simulink model "lqr_linear"  (R2018a)
settings: Solver=FixedStepAuto  StartTime=0.0  StopTime=10  FixedStep=0.001  RelTol=1e-3
values from neighbouring files (symbols this model uses):
  A_dc = [(A_d-B_d*K_d)]    [Project_LQR.m]
  Ac = [(A-B*K)]    [Project_LQR.m]
  B_dc = [B_d]    [Project_LQR.m]
  Bc = [B]    [Project_LQR.m]
  C_dc = [C_d]    [Project_LQR.m]
  Cc = [C]    [Project_LQR.m]
  D_dc = [D_d]    [Project_LQR.m]
  Dc = [D]    [Project_LQR.m]
  Nbar = Nu + K*Nx    [Project_LQR.m]
  Nbar_d = K_d(3)    [Project_LQR.m]
  R_Wheel = 0.04    [Project_LQR.m]    (also in Project_PID.m)
libraries: simulink x5
settings Model: Creator=adios  LastModifiedBy=adios

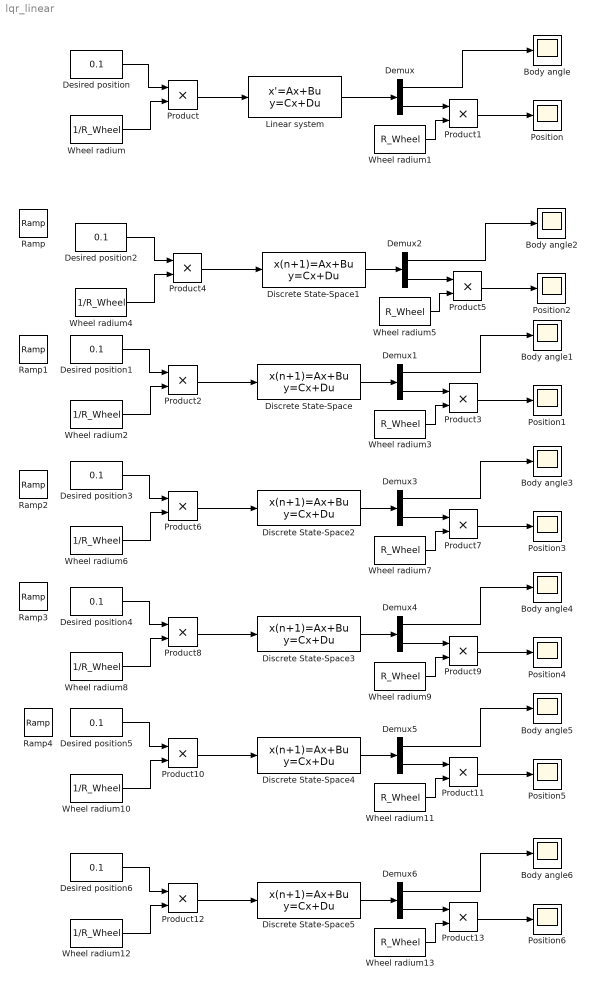
== system lqr_linear ==
  Body angle{,1..6} (7 alike) : Scope
  Demux{,1..6} (7 alike) : Demux  Outputs=2
  Desired position{,1..6} (7 alike) : Constant  Value=0.1
  Discrete State-Space : DiscreteStateSpace  A=A_dc  B=B_dc*Nbar_d  C=C_dc  D=D_dc  InitialCondition=[0 0 0 0]  SampleTime=0.02
  Discrete State-Space1 : DiscreteStateSpace  A=A_dc  B=B_dc*Nbar_d  C=C_dc  D=D_dc  InitialCondition=[0 0 0 0]  SampleTime=0.01
  Discrete State-Space2 : DiscreteStateSpace  A=A_dc  B=B_dc*Nbar_d  C=C_dc  D=D_dc  InitialCondition=[0 0 0 0]  SampleTime=0.04
  Discrete State-Space3 : DiscreteStateSpace  A=A_dc  B=B_dc*Nbar_d  C=C_dc  D=D_dc  InitialCondition=[0 0 0 0]  SampleTime=0.06
  Discrete State-Space4 : DiscreteStateSpace  A=A_dc  B=B_dc*Nbar_d  C=C_dc  D=D_dc  InitialCondition=[0 0 0 0]  SampleTime=0.08
  Discrete State-Space5 : DiscreteStateSpace  A=A_dc  B=B_dc*Nbar_d  C=C_dc  D=D_dc  InitialCondition=[0 0 0 0]  SampleTime=0.1
  Linear system : StateSpace  A=Ac  B=Bc*Nbar  C=Cc  D=Dc  InitialCondition=[0 0 0 0]  ContinuousStateAttributes=['theta' 'theta_dot' 'phi' 'phi_dot']
  Position{,1..6} (7 alike) : Scope
  Product{,1..13} (14 alike) : Product
  Ramp : simulink/Sources/Ramp  slope=0.1  start=0  InitialOutput=0
  Ramp1 : simulink/Sources/Ramp  slope=0.3  start=0  InitialOutput=0
  Ramp2 : simulink/Sources/Ramp  slope=0.5  start=0  InitialOutput=0
  Ramp3 : simulink/Sources/Ramp  slope=0.75  start=0  InitialOutput=0
  Ramp4 : simulink/Sources/Ramp  slope=1  start=0  InitialOutput=0
  Wheel radium{,2,4,6,8,10,12} (7 alike) : Constant  Value=1/R_Wheel
  Wheel radium{1,3,5,7,9,11,13} (7 alike) : Constant  Value=R_Wheel
  wires:
  Linear system/1 -> Demux/1
  Desired position/1 -> Product/1
  Wheel radium/1 -> Product/2
  Product/1 -> Linear system/1
  Demux/1 -> Body angle/1
  Demux/2 -> Product1/1
  Wheel radium1/1 -> Product1/2
  Product1/1 -> Position/1
  Wheel radium2/1 -> Product2/2
  Product2/1 -> Discrete State-Space/1
  Demux1/2 -> Product3/1
  Wheel radium3/1 -> Product3/2
  Demux1/1 -> Body angle1/1
  Product3/1 -> Position1/1
  Discrete State-Space/1 -> Demux1/1
  Wheel radium5/1 -> Product5/2
  Product4/1 -> Discrete State-Space1/1
  Wheel radium4/1 -> Product4/2
  Demux2/1 -> Body angle2/1
  Product5/1 -> Position2/1
  Discrete State-Space1/1 -> Demux2/1
  Demux2/2 -> Product5/1
  Wheel radium7/1 -> Product7/2
  Product6/1 -> Discrete State-Space2/1
  Wheel radium6/1 -> Product6/2
  Demux3/1 -> Body angle3/1
  Product7/1 -> Position3/1
  Discrete State-Space2/1 -> Demux3/1
  Demux3/2 -> Product7/1
  Wheel radium9/1 -> Product9/2
  Product8/1 -> Discrete State-Space3/1
  Wheel radium8/1 -> Product8/2
  Demux4/1 -> Body angle4/1
  Product9/1 -> Position4/1
  Discrete State-Space3/1 -> Demux4/1
  Demux4/2 -> Product9/1
  Product10/1 -> Discrete State-Space4/1
  Product11/1 -> Position5/1
  Wheel radium11/1 -> Product11/2
  Demux5/1 -> Body angle5/1
  Discrete State-Space4/1 -> Demux5/1
  Demux5/2 -> Product11/1
  Wheel radium10/1 -> Product10/2
  Desired position2/1 -> Product4/1
  Desired position1/1 -> Product2/1
  Desired position3/1 -> Product6/1
  Desired position4/1 -> Product8/1
  Desired position5/1 -> Product10/1
  Discrete State-Space5/1 -> Demux6/1
  Demux6/2 -> Product13/1
  Desired position6/1 -> Product12/1
  Product12/1 -> Discrete State-Space5/1
  Product13/1 -> Position6/1
  Wheel radium12/1 -> Product12/2
  Demux6/1 -> Body angle6/1
  Wheel radium13/1 -> Product13/2
